simulink model "ME326_05_Activity4_BonneyCaiden_SimulinkFile"  (R2024b)
settings: Solver=VariableStepAuto  StartTime=0.0  StopTime=15  RelTol=1e-9
undefined symbols (not defined in the file): CrankSlider
settings Model: Creator=jaint  LastModifiedBy=Caide
settings DebuggingCC: UnconnectedInputMsg=warning  UnconnectedOutputMsg=warning  UnconnectedLineMsg=warning
settings ModelReferenceCC: EnableRefExpFcnMdlSchedulingChecks=on
settings RTWCC: GPUComputeCapability=3.5  DLArmComputeVersion=19.05

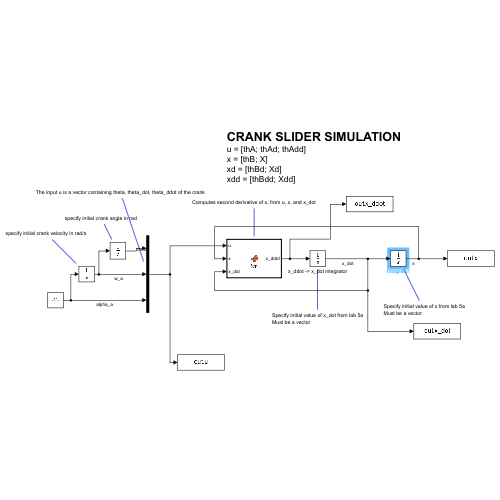
[thumbnail: Simulink's stored preview of the top-level diagram]
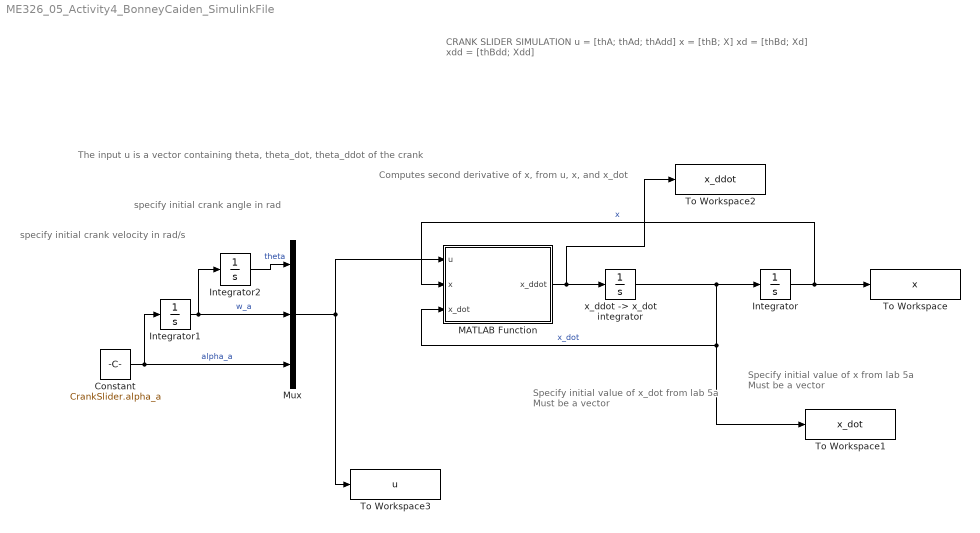
== system ME326_05_Activity4_BonneyCaiden_SimulinkFile ==
  note: CRANK SLIDER SIMULATION
      | u = [thA; thAd; thAdd]
      | x = [thB; X]
      | xd = [thBd; Xd]
      | xdd = [thBdd; Xdd]
  note: specify initial crank velocity in rad/s
  note: specify initial crank angle in rad
  note: The input u is a vector containing theta, theta_dot, theta_ddot of the crank
  note: Specify initial value of x from lab 5a
      | Must be a vector
  note: Computes second derivative of x, from u, x, and x_dot
  note: Specify initial value of x_dot from lab 5a
      | Must be a vector
  Constant : Constant  Value=CrankSlider.alpha_a
  Integrator : Integrator  InitialCondition=CrankSlider.unknowns_vec
  Integrator1 : Integrator  InitialCondition=CrankSlider.w_a
  Integrator2 : Integrator  InitialCondition=CrankSlider.tha_rad
  MATLAB Function : MATLAB Function  TreatAsAtomicUnit=on
  Mux : Mux  Inputs=3
  To Workspace : ToWorkspace  VariableName=x  SampleTime=-1
  To Workspace1 : ToWorkspace  VariableName=x_dot  SampleTime=-1
  To Workspace2 : ToWorkspace  VariableName=x_ddot  SampleTime=-1
  To Workspace3 : ToWorkspace  VariableName=u  SampleTime=-1
  "x_ddot -> x_dot integrator" : Integrator  InitialCondition=CrankSlider.xd
  wires:
  MATLAB Function/1(x_ddot) -> To Workspace2/1, "x_ddot -> x_dot integrator"/1
  "x_ddot -> x_dot integrator"/1 -> To Workspace1/1, MATLAB Function/3(x_dot), Integrator/1  "x_dot"
  Integrator/1 -> MATLAB Function/2(x), To Workspace/1  "x"
  Mux/1 -> To Workspace3/1, MATLAB Function/1(u)
  Integrator1/1 -> Mux/2, Integrator2/1  "w_a"
  Constant/1 -> Mux/3, Integrator1/1  "alpha_a"
  Integrator2/1 -> Mux/1  "theta"

== matlab function ME326_05_Activity4_BonneyCaiden_SimulinkFile/MATLAB Function ==
  data: u input; x input; x_ddot output; x_dot input; CrankSlider parameter
function x_ddot = fcn(u,x,x_dot, CrankSlider)
%% Compute second derivative of the state vector x, based on the input, u
% highlight P, right click on P, change data scope to parameter
% now grabs value for P straight from the workspace

% velocity vector x, and state vecotor x
%Acceleration matrix from lab 3A
%A = [Mech1.r2*Mech1.s2 1;
%     Mech1.r2*Mech1.c2 0];
sA = sin(u(1));
cA = cos(u(1));

thAd_sq = (u(2))^2;
thBd_sq = (x_dot(1))^2;

thAdd = (u(3));

sB = sin(x(1));
cB = cos(x(1));

A = [CrankSlider.L_bc*sB 1;
     CrankSlider.L_bc*cB 0]; 

%b_a = [-Mech1.r1*Mech1.c1*Mech1.th1d^2 - Mech1.r2*Mech1.c2*Mech1.th2d^2;
%        Mech1.r1*Mech1.s1*Mech1.th1d^2 + Mech1.r2*Mech1.s2*Mech1.th2d^2]
b_a = [-CrankSlider.L_ab*cA*thAd_sq - CrankSlider.L_ab*sA*thAdd - CrankSlider.L_bc*cB*thBd_sq;
        CrankSlider.L_ab*sA*thAd_sq - CrankSlider.L_ab*cA*thAdd + CrankSlider.L_bc*sB*thBd_sq];
x_ddot = A\b_a;
